simulink model "model"  (R2024b)
settings: Solver=VariableStepAuto  StartTime=0.0  StopTime=10.0  RelTol=1e-3
values from neighbouring files (symbols this model uses):
  C1 = 100e-6    (= 0.0001)    [Project_script.m]
  C2 = 100e-6    (= 0.0001)    [Project_script.m]
  ki = 2000    [Project_script.m]
  kp1 = 0.01    [Project_script.m]
  kp2 = 0.01    [Project_script.m]
  L = 90e-6    (= 9e-05)    [Project_script.m]
  R1 = 18.432    [Project_script.m]
  Tend = 50e-3    (= 0.05)    [Project_script.m]
  ts = 0.1e-6    (= 1e-07)    [Project_script.m]
  Vi = 24    [Project_script.m]
  voref = 96    [Project_script.m]
undefined symbols (not defined in the file or in its folder): C, R2, R3, R4
libraries: spsSeriesRLCBranchLib x7, spsIdealSwitchLib x5, simulink x4, spsCurrentMeasurementLib x2, spsDiodeLib x2, spsDCVoltageSourceLib x1, spsVoltageMeasurementLib x1, spsPWMGeneratorDCDCLib x1, spspowerguiLib x1
settings Model: Creator=Bogat  LastModifiedBy=Bogat

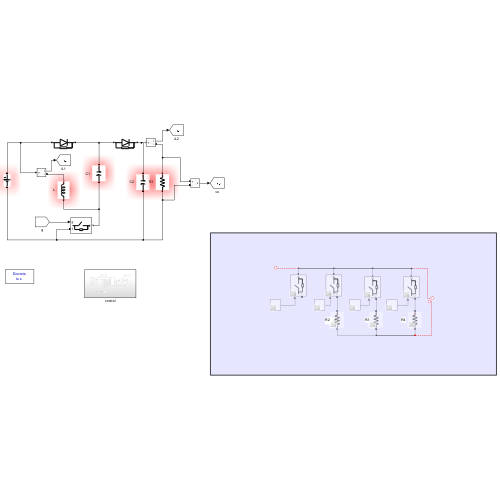
[thumbnail: Simulink's stored preview of the top-level diagram]
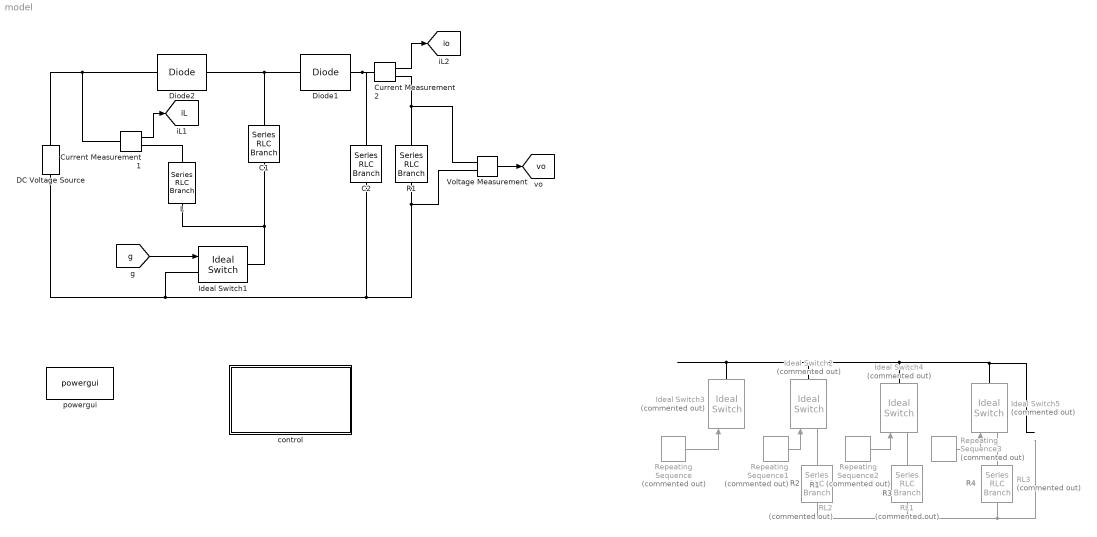
== system model ==
  note: R4
  note: R3
  note: R2
  note: R1
  C1 : spsSeriesRLCBranchLib/Series RLC Branch  LConnTagsString=__new0  RConnTagsString=__new0  BranchType=C  Resistance=1  Inductance=L  SetiL0=on  InitialCurrent=0  Capacitance=C1  Setx0=on  InitialVoltage=0  Measurements=None
  C2 : spsSeriesRLCBranchLib/Series RLC Branch  LConnTagsString=__new0  RConnTagsString=__new0  BranchType=C  Resistance=1  Inductance=L  SetiL0=on  InitialCurrent=0  Capacitance=C2  Setx0=on  InitialVoltage=0  Measurements=None
  Current Measurement1 : spsCurrentMeasurementLib/Current Measurement  PhasorSimulation=off  OutputType=Complex  PSBequivalent=0
  Current Measurement2 : spsCurrentMeasurementLib/Current Measurement  PhasorSimulation=off  OutputType=Complex  PSBequivalent=0
  DC Voltage Source : spsDCVoltageSourceLib/DC Voltage Source  Amplitude=Vi  Measurements=None
  Diode1 : spsDiodeLib/Diode  Ron=0.001  Lon=0  Vf=0.8  IC=0  UseSnubber=0  Rs=500  Cs=250e-9  Measurements=off
  Diode2 : spsDiodeLib/Diode  Ron=0.001  Lon=0  Vf=0.8  IC=0  UseSnubber=0  Rs=500  Cs=250e-9  Measurements=off
  Ideal Switch1 : spsIdealSwitchLib/Ideal Switch  Ron=0.001  Lon=0  IC=0  Rs=1e5  Cs=inf  Measurements=off
  Ideal Switch{2..5} (4 alike) : spsIdealSwitchLib/Ideal Switch  Commented=on  Ron=0.001  Lon=0  IC=0  Rs=1e5  Cs=inf  Measurements=off
  L : spsSeriesRLCBranchLib/Series RLC Branch  LConnTagsString=__new0  RConnTagsString=__new0  BranchType=L  Resistance=1  Inductance=L  SetiL0=on  InitialCurrent=0  Capacitance=1e-6  Setx0=off  InitialVoltage=0  Measurements=None
  R1 : spsSeriesRLCBranchLib/Series RLC Branch  LConnTagsString=__new0  RConnTagsString=__new0  BranchType=R  Resistance=R1  Inductance=L  SetiL0=on  InitialCurrent=0  Capacitance=C  Setx0=on  InitialVoltage=0  Measurements=None
  RL1 : spsSeriesRLCBranchLib/Series RLC Branch  Commented=on  LConnTagsString=__new0  RConnTagsString=__new0  BranchType=R  Resistance=R3  Inductance=L  SetiL0=on  InitialCurrent=0  Capacitance=C  Setx0=on  InitialVoltage=0  Measurements=None
  RL2 : spsSeriesRLCBranchLib/Series RLC Branch  Commented=on  LConnTagsString=__new0  RConnTagsString=__new0  BranchType=R  Resistance=R2  Inductance=L  SetiL0=on  InitialCurrent=0  Capacitance=C  Setx0=on  InitialVoltage=0  Measurements=None
  RL3 : spsSeriesRLCBranchLib/Series RLC Branch  Commented=on  LConnTagsString=__new0  RConnTagsString=__new0  BranchType=R  Resistance=R4  Inductance=L  SetiL0=on  InitialCurrent=0  Capacitance=C  Setx0=on  InitialVoltage=0  Measurements=None
  Repeating Sequence : simulink/Sources/Repeating Sequence  Commented=on  rep_seq_t=[0 0.2*Tend 0.2*Tend+ts Tend]  rep_seq_y=[1 1 0 0]
  Repeating Sequence1 : simulink/Sources/Repeating Sequence  Commented=on  rep_seq_t=[0 0.2*Tend 0.2*Tend+ts 0.4*Tend 0.4*Tend+ts Tend]  rep_seq_y=[0 0 1 1 0 0]
  Repeating Sequence2 : simulink/Sources/Repeating Sequence  Commented=on  rep_seq_t=[0 0.4*Tend 0.4*Tend+ts 0.6*Tend 0.6*Tend+ts Tend]  rep_seq_y=[0 0 1 1 0 0]
  Repeating Sequence3 : simulink/Sources/Repeating Sequence  Commented=on  rep_seq_t=[0 0.6*Tend 0.6*Tend+ts Tend]  rep_seq_y=[0 0 1 1]
  Voltage Measurement : spsVoltageMeasurementLib/Voltage Measurement  PhasorSimulation=off  OutputType=Complex  PSBequivalent=0
  control : Subsystem
  powergui : spspowerguiLib/powergui  Priority=1  SimulationMode=Discrete  SampleTime=ts  frequency=60  Iterations=50  frequencyindice=0  Pbase=100e6  ErrMax=1e-4  UnitsV=kV  UnitsW=MW  buscounter=0  FunctionMessages=off  echomessages=off  EnableUseOfTLC=off  CurrentSourceSwitches=off  DisableSnubberDevices=off  DisableRonSwitches=off  DisableVfSwitches=off  DisplayEquations=off  AutomaticDiscreteSolvers=off  SolverType=Tustin/Backward Euler (TBE)  Interpol=off  ExternalGateDelay=off  methode=off  Ts=100  x0status=blocks  SPID=on  SwTol=0  HookPort=off  NonlinearTolerance=1e-4  nMaxIteration=100  ContinueOnMaxIteration=off  RestoreLinks=warning  ResistiveCurrentMeasurement=off  Frange=[0:2:500]  Ylog=off  Xlog=on  ShowGrid=off  save=off  variable=ZData  structure=0  ZoomFFT=off  StartTime=0.0  cycles=1  DisplayStyle=1  fundamental=60  FreqAxis=off  MaxFrequency=1000  frequencyindicesteady=1  RmsSteady=1  display=off
  tag scope: iL=global, io=global, vo=global
  wires:
  Voltage Measurement/1 -> [vo]
  [g] -> Ideal Switch1/1
  Current Measurement1/1 -> [iL]
  Current Measurement2/1 -> [io]
  Repeating Sequence2/1 -> Ideal Switch4/1
  Repeating Sequence1/1 -> Ideal Switch2/1
  Repeating Sequence3/1 -> Ideal Switch5/1
  Repeating Sequence/1 -> Ideal Switch3/1
  connections:
  Diode1/RConn1 -- C2/LConn1 -- Current Measurement2/LConn1
  Ideal Switch1/LConn1 -- DC Voltage Source/LConn1 -- Voltage Measurement/LConn2 -- R1/RConn1 -- C2/RConn1
  C1/LConn1 -- Diode2/RConn1 -- Diode1/LConn1
  Current Measurement1/RConn1 -- L/LConn1
  Ideal Switch3/RConn1 -- Ideal Switch2/RConn1 -- Ideal Switch4/RConn1 -- Ideal Switch5/RConn1
  RL2/RConn1 -- RL3/RConn1 -- RL1/RConn1
  RL1/LConn1 -- Ideal Switch4/LConn1
  RL2/LConn1 -- Ideal Switch2/LConn1
  RL3/LConn1 -- Ideal Switch5/LConn1
  Current Measurement2/RConn1 -- R1/LConn1 -- Voltage Measurement/LConn1
  Ideal Switch1/RConn1 -- C1/RConn1 -- L/RConn1
  DC Voltage Source/RConn1 -- Diode2/LConn1 -- Current Measurement1/LConn1

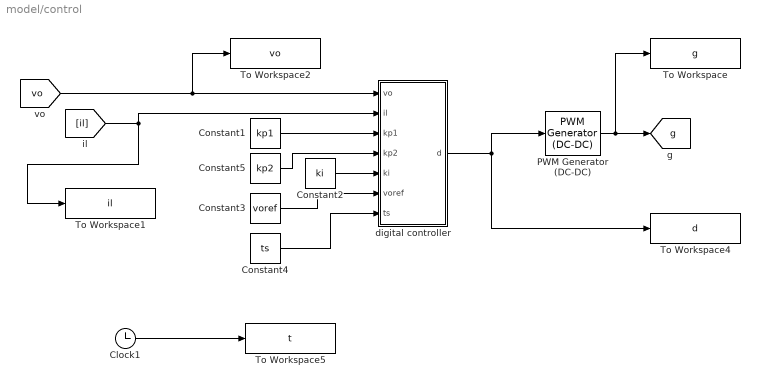
== system model/control ==
  Clock1 : Clock
  Constant1 : Constant  Value=kp1
  Constant2 : Constant  Value=ki
  Constant3 : Constant  Value=voref
  Constant4 : Constant  Value=ts
  Constant5 : Constant  Value=kp2
  PWM Generator (DC-DC) : spsPWMGeneratorDCDCLib/PWM Generator (DC-DC)  Fsw=fs  Ts=ts
  To Workspace : ToWorkspace  VariableName=g  SampleTime=ts
  To Workspace1 : ToWorkspace  VariableName=il  SampleTime=ts
  To Workspace2 : ToWorkspace  VariableName=vo  SampleTime=ts
  To Workspace4 : ToWorkspace  VariableName=d  SampleTime=ts
  To Workspace5 : ToWorkspace  VariableName=t  SampleTime=ts
  digital controller : MATLAB Function  TreatAsAtomicUnit=on
  tag scope: g=global
  wires:
  digital controller/1(d) -> PWM Generator (DC-DC)/1, To Workspace4/1
  [vo] -> To Workspace2/1, digital controller/1(vo)
  PWM Generator (DC-DC)/1 -> [g], To Workspace/1
  Clock1/1 -> To Workspace5/1
  Constant1/1 -> digital controller/3(kp1)
  Constant2/1 -> digital controller/5(ki)
  Constant3/1 -> digital controller/6(voref)
  Constant4/1 -> digital controller/7(ts)
  Constant5/1 -> digital controller/4(kp2)
  [il] -> To Workspace1/1, digital controller/2(il)

== matlab function model/control/digital controller ==
  data: vo input; il input; kp1 input; kp2 input; ki input; voref input; d output; ts input
function d = fcn(vo,il,kp1,kp2,ki,voref,ts)

persistent int_1
if isempty(int_1)
    int_1=0;
end

int=int_1+ki*ts*(voref-vo);
ilref=kp1*(voref-vo)+int;

d=kp2*(ilref-il);

if (d>1)
    int=int_1; % anti-windup
    d=1;
end
if (d<0)
    int=int_1; % anti-windup
    d=0;
end
int_1=int;
